simulink model "keg_mealy"  (R2015a)
settings: Solver=ode3  StartTime=0.0  StopTime=300  RelTol=1e-3
undefined symbols (not defined in the file): sigbuilder_block
settings Model: Creator=lenovo  LastModifiedBy=lenovo

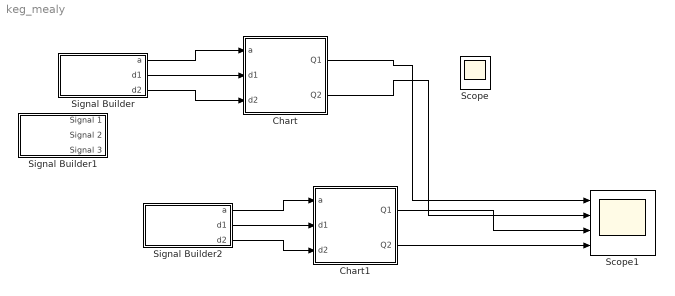
== system keg_mealy ==
  Chart : Stateflow chart  TreatAsAtomicUnit=on
  Chart1 : Stateflow chart  TreatAsAtomicUnit=on
  Scope : Scope  NumInputPorts=2
      settings: YMin=-5~-5  YMax=5~5
  Scope1 : Scope  NumInputPorts=4
      settings: YMin=-5~-5~-5~-5  YMax=5~5~5~5
  Signal Builder : Subsystem  Tag=STV Subsys  LoadFcn=sigbuilder_block('load');  StartFcn=sigbuilder_block('start');  StopFcn=sigbuilder_block('stop');  ClipboardFcn=sigbuilder_block('clipboard');  mask(Sigbuilder block){}
      mask help: Simulink:masks:SigbuilderBlock_MD
      mask init:
      | if ~strcmp(get_param(bdroot(gcbh),'SimulationStatus'),'stopped') tuvar = sigbuilder_block('maskInit'); end
      settings: CopyFcn=sigbuilder_block('copy');  DeleteFcn=sigbuilder_block('delete');  ModelCloseFcn=sigbuilder_block('modelClose');  PreSaveFcn=sigbuilder_block('preSave');  PauseFcn=sigbuilder_block('pause');  ContinueFcn=sigbuilder_block('continue');  NameChangeFcn=sigbuilder_block('namechange');  OpenFcn=sigbuilder_block('open',[437.6 199.2 550.4 400 ]);  CloseFcn=sigbuilder_block('close');
      mask Display: plot(0, 0, 100, 100,[2, 2, 32, 32, 2], [68, 8, 8, 68, 68],[32, 2], [38, 38], [32, 19, 2],[53, 60, 44], [32, 17, 17, 2],[16, 16, 31, 31]);txt = getActiveGroup(gcbh);text(2, 100, txt,'verticalAlignment', 'top');
  Signal Builder1 : Subsystem  Tag=STV Subsys  LoadFcn=sigbuilder_block('load');  StartFcn=sigbuilder_block('start');  StopFcn=sigbuilder_block('stop');  ClipboardFcn=sigbuilder_block('clipboard');  mask(Sigbuilder block){}
      mask help: Simulink:masks:SigbuilderBlock_MD
      mask init:
      | if ~strcmp(get_param(bdroot(gcbh),'SimulationStatus'),'stopped') tuvar = sigbuilder_block('maskInit'); end
      settings: CopyFcn=sigbuilder_block('copy');  DeleteFcn=sigbuilder_block('delete');  ModelCloseFcn=sigbuilder_block('modelClose');  PreSaveFcn=sigbuilder_block('preSave');  PauseFcn=sigbuilder_block('pause');  ContinueFcn=sigbuilder_block('continue');  NameChangeFcn=sigbuilder_block('namechange');  OpenFcn=sigbuilder_block('open',[198.75 94.5 550.5 399.75 ]);  CloseFcn=sigbuilder_block('close');
      mask Display: plot(0, 0, 100, 100,[2, 2, 32, 32, 2], [68, 8, 8, 68, 68],[32, 2], [38, 38], [32, 19, 2],[53, 60, 44], [32, 17, 17, 2],[16, 16, 31, 31]);txt = getActiveGroup(gcbh);text(2, 100, txt,'verticalAlignment', 'top');
  Signal Builder2 : Subsystem  Tag=STV Subsys  LoadFcn=sigbuilder_block('load');  StartFcn=sigbuilder_block('start');  StopFcn=sigbuilder_block('stop');  ClipboardFcn=sigbuilder_block('clipboard');  mask(Sigbuilder block){}
      mask help: Simulink:masks:SigbuilderBlock_MD
      mask init:
      | if ~strcmp(get_param(bdroot(gcbh),'SimulationStatus'),'stopped') tuvar = sigbuilder_block('maskInit'); end
      settings: CopyFcn=sigbuilder_block('copy');  DeleteFcn=sigbuilder_block('delete');  ModelCloseFcn=sigbuilder_block('modelClose');  PreSaveFcn=sigbuilder_block('preSave');  PauseFcn=sigbuilder_block('pause');  ContinueFcn=sigbuilder_block('continue');  NameChangeFcn=sigbuilder_block('namechange');  OpenFcn=sigbuilder_block('open',[437.6 199.2 550.4 400 ]);  CloseFcn=sigbuilder_block('close');
      mask Display: plot(0, 0, 100, 100,[2, 2, 32, 32, 2], [68, 8, 8, 68, 68],[32, 2], [38, 38], [32, 19, 2],[53, 60, 44], [32, 17, 17, 2],[16, 16, 31, 31]);txt = getActiveGroup(gcbh);text(2, 100, txt,'verticalAlignment', 'top');
  wires:
  Chart/1(Q1) -> Scope1/1
  Chart/2(Q2) -> Scope1/2
  Chart1/1(Q1) -> Scope1/3
  Signal Builder2/1(a) -> Chart1/1(a)
  Signal Builder2/2(d1) -> Chart1/2(d1)
  Signal Builder2/3(d2) -> Chart1/3(d2)
  Chart1/2(Q2) -> Scope1/4
  Signal Builder/3(d2) -> Chart/3(d2)
  Signal Builder/2(d1) -> Chart/2(d1)
  Signal Builder/1(a) -> Chart/1(a)

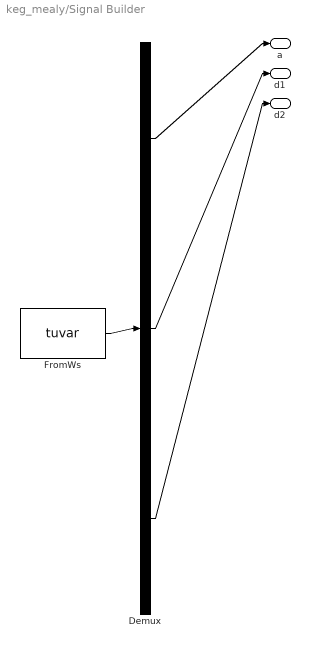
== system keg_mealy/Signal Builder ==
  Demux : Demux  Tag=STV Demux  Outputs=3
  FromWs : FromWorkspace  Tag=STV FromWs  VariableName=tuvar  SampleTime=0
      SigBuilderData=|
      | common.afterFinalStr = 'Extrapolate'
      | common.sampleTime = 0
      | dataSet.timeRange = [0 300]
      | dataSet.name = 'Group 1'
      | sbobj.Groups.Name = 'Group 1'
      | sbobj.Groups.Signals(1).Name = 'a'
      | sbobj.Groups.Signals(1).XData = [0 30 30 35.5 35.5 90 90 96.5 96.5 150 150 155.5 155.5 210 210 217.5 217.5 270 270 278.5 278.5 300]
      | sbobj.Groups.Signals(1).YData = [0 0 1 1 0 0 1 1 0 0 1 1 0 0 1 1 0 0 1 1 0 0]
      | sbobj.Groups.Signals(2).Name = 'd1'
      | sbobj.Groups.Signals(2).XData = [0 25 50 50 57.5 57.5 100 100 106 106 155 155 160.5 160.5 212 212 219.5 219.5 274.5 274.5 280 280 300]
      | sbobj.Groups.Signals(2).YData = [0 0 0 1 1 0 0 1 1 0 0 1 1 0 0 1 1 0 0 1 1 0 0]
      | sbobj.Groups.Signals(3).Name = 'd2'
      | sbobj.Groups.Signals(3).XData = [0 25 69 69 76 76 121 121 128.5 128.5 149 149 153.5 153.5 202.5 202.5 206.5 206.5 265 265 270.5 270.5 300]
      | sbobj.Groups.Signals(3).YData = [0 0 0 1 1 0 0 1 1 0 0 1 1 0 0 1 1 0 0 1 1 0 0]
      | sbobj.Groups.TimeRange = [0 300]
  a : Outport  Tag=STV Outport
  d1 : Outport  Tag=STV Outport  Port=2
  d2 : Outport  Tag=STV Outport  Port=3
  wires:
  Demux/1 -> a/1
  Demux/2 -> d1/1
  Demux/3 -> d2/1
  FromWs/1 -> Demux/1

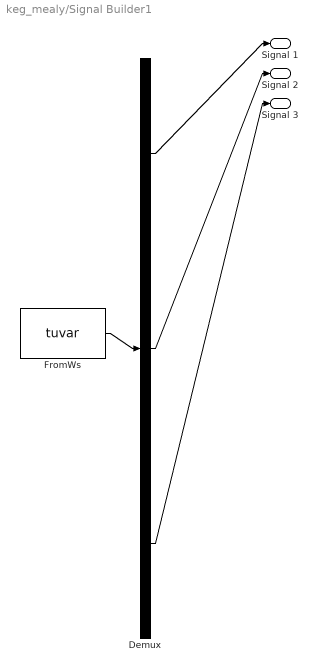
== system keg_mealy/Signal Builder1 ==
  Demux : Demux  Tag=STV Demux  Outputs=3
  FromWs : FromWorkspace  Tag=STV FromWs  VariableName=tuvar  SampleTime=0
      SigBuilderData=|
      | common.afterFinalStr = 'Extrapolate'
      | common.sampleTime = 0
      | dataSet.timeRange = [0 600]
      | dataSet.name = 'Group 1'
      | sbobj.Groups.Name = 'Group 1'
      | sbobj.Groups.Signals(1).Name = 'Signal 1'
      | sbobj.Groups.Signals(1).XData = [0 7 7 42 42 47 47 100 100 106 106 150 150 155 155 200 200 203 203 250 250 252 252 300 300 304 304 350 350 354 354 400 400 403 403 450 450 454 454 500 500 505 505 550 550 552 552 600]
      | sbobj.Groups.Signals(1).YData = [1 1 0 0 1 1 0 0 1 1 0 0 1 1 0 0 1 1 0 0 1 1 0 0 1 1 0 0 1 1 0 0 1 1 0 0 1 1 0 0 1 1 0 0 1 1 0 0]
      | sbobj.Groups.Signals(2).Name = 'Signal 2'
      | sbobj.Groups.Signals(2).XData = [0 50 74 74 80 80 134 134 141 141 231 231 235 235 321 321 324 324 433 433 440 440 600]
      | sbobj.Groups.Signals(2).YData = [0 0 0 1 1 0 0 1 1 0 0 1 1 0 0 1 1 0 0 1 1 0 0]
      | sbobj.Groups.Signals(3).Name = 'Signal 3'
      | sbobj.Groups.Signals(3).XData = [0 25 50 75 105 105 111 111 150 175 196 196 205 205 274 287 300 325 350 375 400 400 409 409 454 475 500 500 505 505 550 575 600]
      | sbobj.Groups.Signals(3).YData = [0 0 0 0 0 1 1 0 0 0 0 1 1 0 0 0 0 0 0 0 0 1 1 0 0 0 0 1 1 0 0 0 0]
      | sbobj.Groups.TimeRange = [0 600]
  Signal 1 : Outport  Tag=STV Outport
  Signal 2 : Outport  Tag=STV Outport  Port=2
  Signal 3 : Outport  Tag=STV Outport  Port=3
  wires:
  Demux/1 -> Signal 1/1
  Demux/2 -> Signal 2/1
  Demux/3 -> Signal 3/1
  FromWs/1 -> Demux/1

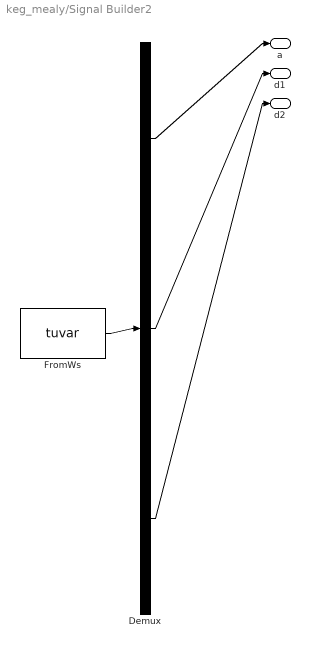
== system keg_mealy/Signal Builder2 ==
  Demux : Demux  Tag=STV Demux  Outputs=3
  FromWs : FromWorkspace  Tag=STV FromWs  VariableName=tuvar  SampleTime=0
      SigBuilderData=|
      | common.afterFinalStr = 'Extrapolate'
      | common.sampleTime = 0
      | dataSet.timeRange = [0 300]
      | dataSet.name = 'Group 1'
      | sbobj.Groups.Name = 'Group 1'
      | sbobj.Groups.Signals(1).Name = 'a'
      | sbobj.Groups.Signals(1).XData = [0 30 30 40 40 90 90 100 100 150 150 160 160 210 210 220 220 270 270 280 280 300]
      | sbobj.Groups.Signals(1).YData = [0 0 1 1 0 0 1 1 0 0 1 1 0 0 1 1 0 0 1 1 0 0]
      | sbobj.Groups.Signals(2).Name = 'd1'
      | sbobj.Groups.Signals(2).XData = [0 25 50 50 75 75 100 100 125 125 150 150 175 175 200 200 225 225 250 250 275 275 300]
      | sbobj.Groups.Signals(2).YData = [0 0 0 1 1 0 0 1 1 0 0 1 1 0 0 1 1 0 0 1 1 0 0]
      | sbobj.Groups.Signals(3).Name = 'd2'
      | sbobj.Groups.Signals(3).XData = [0 25 35.5 45.5 86 86 94 94 154.5 154.5 161.5 161.5 182.5 182.5 192.5 192.5 231 231 275 275 300]
      | sbobj.Groups.Signals(3).YData = [0 0 0 0 0 1 1 0 0 1 1 0 0 1 1 0 0 1 1 0 0]
      | sbobj.Groups.TimeRange = [0 300]
  a : Outport  Tag=STV Outport
  d1 : Outport  Tag=STV Outport  Port=2
  d2 : Outport  Tag=STV Outport  Port=3
  wires:
  Demux/1 -> a/1
  Demux/2 -> d1/1
  Demux/3 -> d2/1
  FromWs/1 -> Demux/1

== stateflow chart keg_mealy/Chart1 ==
  settings: stateMachineType=MOORE_MACHINE
  state 01
    Q1=0;
    Q2=1;
  state 00
    Q1=0;
    Q2=0;
  state 21
    Q1=2;
    Q2=1;
  state 11
    Q1=1;
    Q2=1;
  state 10
    Q1=1;
    Q2=0;
  01 -> 00 [order 2] : [a==0&d2==1]
  11 -> 10 [order 1] : [a==1&d1==1&d2==1]
  (default) -> 00
  10 -> 01 [order 1] : [a==0&d1==1]
  00 -> 10 : [a==1]
  01 -> 11 [order 3] : [a==1&d1==1d2==0]
  11 -> 21 [order 2] : [a==1&d1==1&d2==0]
  01 -> 00 [order 1] : [a==0&d1==1&d2==1]
  01 -> 10 [order 4] : [a==1&d1==1&d2==1]
  21 -> 01 : [d2==1]
  10 -> 21 [order 2] : [d2==0]
  data: a input; d1 input; d2 input; Q1 output; Q2 output

== stateflow chart keg_mealy/Chart ==
  settings: stateMachineType=MEALY_MACHINE
  state 01
  state 00
  state 21
  state 11
  state 10
  11 -> 10 [order 1] : [d2==1]{Q1=1;Q2=0}
  (default) -> 00
  11 -> 21 [order 3] : [a==1&d1==1&d2==0]{Q1=2;Q2=1}
  10 -> 01 [order 1] : [d1==1]{Q1=0;Q2=1}
  00 -> 10 : [a==1]{Q1=1;Q2=0}
  01 -> 11 [order 2] : [a==1]{Q1=1;Q2=1}
  21 -> 11 [order 2] : [a==1&d2==1]{Q1=1;Q2=1}
  01 -> 10 [order 3] : [a==1&d2==1]{Q1=1;Q2=0}
  10 -> 10 [order 2] : [a==1]{Q1=1;Q2=0}
  01 -> 00 [order 1] : [a==0&d2==1]{Q1=0;Q2=0}
  21 -> 01 [order 1] : [d2==1&a==0]{Q1=0;Q2=1}
  11 -> 11 [order 2] : [a==1]{Q1=1;Q2=1}
  data: a input; d1 input; d2 input; Q1 output; Q2 output
